simulink model "SystemComposer"  (R2023a)
settings: Solver=VariableStepAuto  StartTime=0.0  StopTime=10.0  RelTol=1e-3
settings Model: Creator=ycheb  LastModifiedBy=ycheb

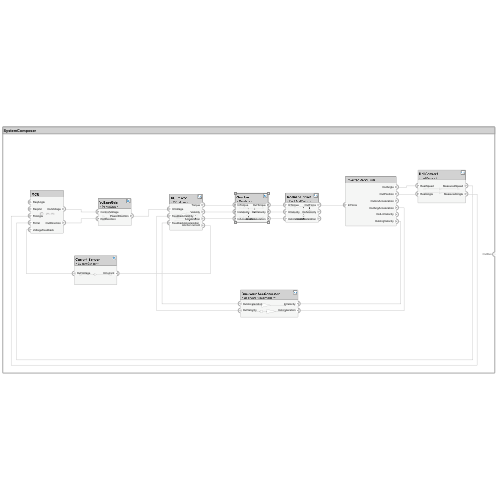
[thumbnail: Simulink's stored preview of the top-level diagram]
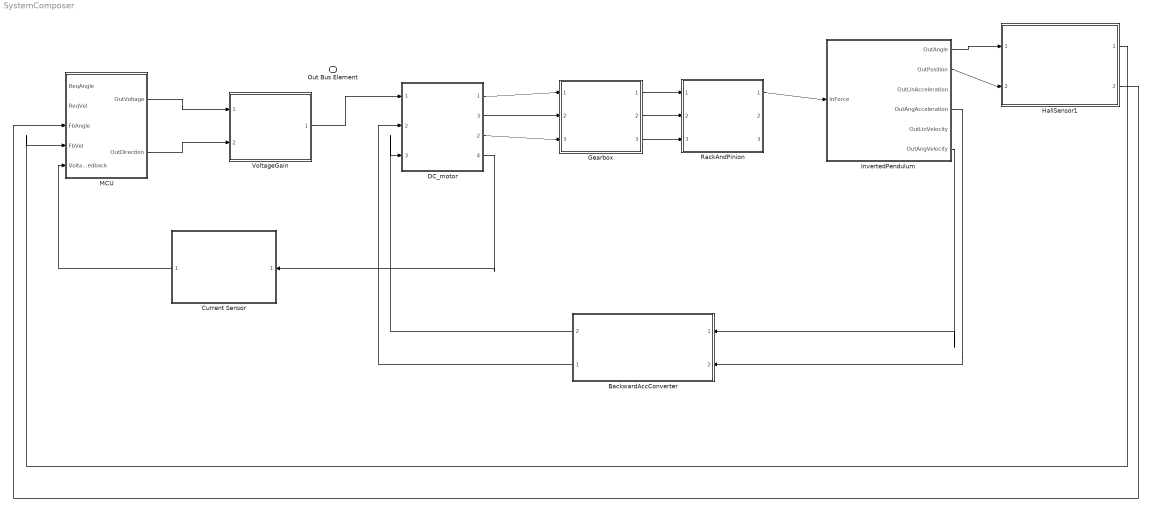
== system SystemComposer ==
  BackwardAccConverter : Subsystem  ReferencedSubsystem=BackwardAccConverter  i_gearbox=0  i_rail=0
      settings: PortSchema="{\"entries\":[{\"content\":{\"headerSize\":26,\"margin\":15,\"minimumSpacing\":25,\"sides\":[{\"content\":{\"connectorIds\":[\"Out2\",\"Out1\"]},\"type\":\"ConnectorPlacement.EquallySpacedRectSide\",\"uuid\":\"4580426d-ccc6-43cc-b0f4-903a280dd54a\"},{\"content\":{\"connectorIds\":[\"In1\",\"In2\"],\"side\":\"RIGHT\"},\"type\":\"ConnectorPlacement.EquallySpacedRectSide\",\"uuid\":\"b139a8af-3718-4301-b11f-f92378786662\"},{\"content\":{\"side\":\"TOP\"},\"type\":\"ConnectorPlacement.EquallySpacedRectSide\",\"uuid\":\"6cad6356-70f4-40af-85cc-1c4aec951e56\"}]},\"type\":\"ConnectorPlacement.EquallySpacedConnector\",\"uuid\":\"b6d7cb52-78ef-4ff8-a29a-dce0cd7ecabe\"}],\"packageUris\":[\"http://schema.mathworks.com/mf0/Connector/R2020b\"],\"version\":\"1.0\"}"
  Current Sensor : Subsystem  ReferencedSubsystem=CurrentSensor  R=0
      settings: PortSchema="{\"entries\":[{\"content\":{\"headerSize\":26,\"margin\":15,\"minimumSpacing\":25,\"sides\":[{\"content\":{\"connectorIds\":[\"Out1\"]},\"type\":\"ConnectorPlacement.EquallySpacedRectSide\",\"uuid\":\"1189f8f4-25dd-42ea-848e-97e302516e0e\"},{\"content\":{\"connectorIds\":[\"In1\"],\"side\":\"RIGHT\"},\"type\":\"ConnectorPlacement.EquallySpacedRectSide\",\"uuid\":\"7a8b9a95-7ade-4c5d-b769-aa776a1a8446\"},{\"content\":{\"side\":\"TOP\"},\"type\":\"ConnectorPlacement.EquallySpacedRectSide\",\"uuid\":\"ebb76304-2a77-452c-a318-4e5ff347d389\"}]},\"type\":\"ConnectorPlacement.EquallySpacedConnector\",\"uuid\":\"42e58dc7-ce24-4261-ad85-d72d6d49920a\"}],\"packageUris\":[\"http://schema.mathworks.com/mf0/Connector/R2020b\"],\"version\":\"1.0\"}"
  DC_motor : Subsystem  ReferencedSubsystem=DC_Motor  L=1  R=0  kw=0  km=0  J_motor=0  vis_friction_coef_motor=0
      settings: PortSchema="{\"entries\":[{\"content\":{\"headerSize\":26,\"margin\":15,\"minimumSpacing\":25,\"sides\":[{\"content\":{\"connectorIds\":[\"In1\",\"In2\",\"In3\"]},\"type\":\"ConnectorPlacement.EquallySpacedRectSide\",\"uuid\":\"195a28a2-a901-462e-beb9-5fc63a42afb4\"},{\"content\":{\"connectorIds\":[\"Out1\",\"Out3\",\"Out2\",\"Out4\"],\"side\":\"RIGHT\"},\"type\":\"ConnectorPlacement.EquallySpacedRectSide\",\"uuid\":\"0ccc545b-fa97-4bbe-bc7a-d14d9e9ad049\"},{\"content\":{\"side\":\"TOP\"},\"type\":\"ConnectorPlacement.EquallySpacedRectSide\",\"uuid\":\"58be0038-e581-4079-a9e4-051b8ced1df8\"}]},\"type\":\"ConnectorPlacement.EquallySpacedConnector\",\"uuid\":\"5194a1e3-6e8a-4730-ada4-e791e93f85f2\"}],\"packageUris\":[\"http://schema.mathworks.com/mf0/Connector/R2020b\"],\"version\":\"1.0\"}"
  Gearbox : Subsystem  ReferencedSubsystem=Gearbox  i=100  J_gear=2,4*10^-6  vis_friction_coef_gear=0.05
      settings: PortSchema="{\"entries\":[{\"content\":{\"headerSize\":26,\"margin\":15,\"minimumSpacing\":25,\"sides\":[{\"content\":{\"connectorIds\":[\"In1\",\"In2\",\"In3\"]},\"type\":\"ConnectorPlacement.EquallySpacedRectSide\",\"uuid\":\"4580426d-ccc6-43cc-b0f4-903a280dd54a\"},{\"content\":{\"connectorIds\":[\"Out1\",\"Out2\",\"Out3\"],\"side\":\"RIGHT\"},\"type\":\"ConnectorPlacement.EquallySpacedRectSide\",\"uuid\":\"b139a8af-3718-4301-b11f-f92378786662\"},{\"content\":{\"side\":\"TOP\"},\"type\":\"ConnectorPlacement.EquallySpacedRectSide\",\"uuid\":\"6cad6356-70f4-40af-85cc-1c4aec951e56\"}]},\"type\":\"ConnectorPlacement.EquallySpacedConnector\",\"uuid\":\"b6d7cb52-78ef-4ff8-a29a-dce0cd7ecabe\"}],\"packageUris\":[\"http://schema.mathworks.com/mf0/Connector/R2020b\"],\"version\":\"1.0\"}"
  HallSensor1 : Subsystem  ReferencedSubsystem=HallSensor
      settings: PortSchema="{\"entries\":[{\"content\":{\"headerSize\":26,\"margin\":15,\"minimumSpacing\":25,\"sides\":[{\"content\":{\"connectorIds\":[\"In1\",\"In2\"]},\"type\":\"ConnectorPlacement.EquallySpacedRectSide\",\"uuid\":\"d9e7e576-5a9b-43ea-8997-3be0b54a9a08\"},{\"content\":{\"connectorIds\":[\"Out1\",\"Out2\"],\"side\":\"RIGHT\"},\"type\":\"ConnectorPlacement.EquallySpacedRectSide\",\"uuid\":\"b8220865-259e-4734-b379-48897555c59f\"},{\"content\":{\"side\":\"TOP\"},\"type\":\"ConnectorPlacement.EquallySpacedRectSide\",\"uuid\":\"b1d688a9-3b35-4d53-b88e-55ef185f4acb\"}]},\"type\":\"ConnectorPlacement.EquallySpacedConnector\",\"uuid\":\"78f6d3ed-99d0-444d-b6d6-a0dd90eae3cb\"}],\"packageUris\":[\"http://schema.mathworks.com/mf0/Connector/R2020b\"],\"version\":\"1.0\"}"
  InvertedPendulum : Subsystem
      settings: PortSchema="{\"entries\":[{\"content\":{\"headerSize\":26,\"margin\":15,\"minimumSpacing\":25,\"sides\":[{\"content\":{\"connectorIds\":[\"In1\"]},\"type\":\"ConnectorPlacement.EquallySpacedRectSide\",\"uuid\":\"d9e7e576-5a9b-43ea-8997-3be0b54a9a08\"},{\"content\":{\"connectorIds\":[\"Out5\",\"Out6\",\"Out1\",\"Out2\",\"Out3\",\"Out4\"],\"side\":\"RIGHT\"},\"type\":\"ConnectorPlacement.EquallySpacedRectSide\",\"uuid\":\"b8220865-259e-4734-b379-48897555c59f\"},{\"content\":{\"side\":\"TOP\"},\"type\":\"ConnectorPlacement.EquallySpacedRectSide\",\"uuid\":\"b1d688a9-3b35-4d53-b88e-55ef185f4acb\"}]},\"type\":\"ConnectorPlacement.EquallySpacedConnector\",\"uuid\":\"78f6d3ed-99d0-444d-b6d6-a0dd90eae3cb\"}],\"packageUris\":[\"http://schema.mathworks.com/mf0/Connector/R2020b\"],\"version\":\"1.0\"}"
  MCU : Subsystem
      settings: PortSchema="{\"entries\":[{\"content\":{\"headerSize\":26,\"margin\":15,\"minimumSpacing\":25,\"sides\":[{\"content\":{\"connectorIds\":[\"In1\",\"In2\",\"In4\",\"In3\",\"In5\"]},\"type\":\"ConnectorPlacement.EquallySpacedRectSide\",\"uuid\":\"d9e7e576-5a9b-43ea-8997-3be0b54a9a08\"},{\"content\":{\"connectorIds\":[\"Out2\",\"Out1\"],\"side\":\"RIGHT\"},\"type\":\"ConnectorPlacement.EquallySpacedRectSide\",\"uuid\":\"b8220865-259e-4734-b379-48897555c59f\"},{\"content\":{\"side\":\"TOP\"},\"type\":\"ConnectorPlacement.EquallySpacedRectSide\",\"uuid\":\"b1d688a9-3b35-4d53-b88e-55ef185f4acb\"}]},\"type\":\"ConnectorPlacement.EquallySpacedConnector\",\"uuid\":\"78f6d3ed-99d0-444d-b6d6-a0dd90eae3cb\"}],\"packageUris\":[\"http://schema.mathworks.com/mf0/Connector/R2020b\"],\"version\":\"1.0\"}"
  RackAndPinion : Subsystem  ReferencedSubsystem=RackAndPinion  I_rail=0  m_rail=0  k_visco=0  i=0
      settings: PortSchema="{\"entries\":[{\"content\":{\"headerSize\":26,\"margin\":15,\"minimumSpacing\":25,\"sides\":[{\"content\":{\"connectorIds\":[\"In1\",\"In2\",\"In3\"]},\"type\":\"ConnectorPlacement.EquallySpacedRectSide\",\"uuid\":\"4580426d-ccc6-43cc-b0f4-903a280dd54a\"},{\"content\":{\"connectorIds\":[\"Out1\",\"Out2\",\"Out3\"],\"side\":\"RIGHT\"},\"type\":\"ConnectorPlacement.EquallySpacedRectSide\",\"uuid\":\"b139a8af-3718-4301-b11f-f92378786662\"},{\"content\":{\"side\":\"TOP\"},\"type\":\"ConnectorPlacement.EquallySpacedRectSide\",\"uuid\":\"6cad6356-70f4-40af-85cc-1c4aec951e56\"}]},\"type\":\"ConnectorPlacement.EquallySpacedConnector\",\"uuid\":\"b6d7cb52-78ef-4ff8-a29a-dce0cd7ecabe\"}],\"packageUris\":[\"http://schema.mathworks.com/mf0/Connector/R2020b\"],\"version\":\"1.0\"}"
  VoltageGain : Subsystem  ReferencedSubsystem=PowerGain  max_output_voltage=0  gain=0
      settings: PortSchema="{\"entries\":[{\"content\":{\"headerSize\":26,\"margin\":15,\"minimumSpacing\":25,\"sides\":[{\"content\":{\"connectorIds\":[\"In1\",\"In2\"]},\"type\":\"ConnectorPlacement.EquallySpacedRectSide\",\"uuid\":\"d9e7e576-5a9b-43ea-8997-3be0b54a9a08\"},{\"content\":{\"connectorIds\":[\"Out1\"],\"side\":\"RIGHT\"},\"type\":\"ConnectorPlacement.EquallySpacedRectSide\",\"uuid\":\"b8220865-259e-4734-b379-48897555c59f\"},{\"content\":{\"side\":\"TOP\"},\"type\":\"ConnectorPlacement.EquallySpacedRectSide\",\"uuid\":\"b1d688a9-3b35-4d53-b88e-55ef185f4acb\"}]},\"type\":\"ConnectorPlacement.EquallySpacedConnector\",\"uuid\":\"78f6d3ed-99d0-444d-b6d6-a0dd90eae3cb\"}],\"packageUris\":[\"http://schema.mathworks.com/mf0/Connector/R2020b\"],\"version\":\"1.0\"}"
  Out Bus Element : Outport  PortName=OutBus
  wires:
  InvertedPendulum/6(OutPosition) -> HallSensor1/2
  InvertedPendulum/5(OutAngle) -> HallSensor1/1
  HallSensor1/2 -> MCU/4(FbAngle)
  HallSensor1/1 -> MCU/3(FbVel)
  MCU/2(OutVoltage) -> VoltageGain/1
  MCU/1(OutDirection) -> VoltageGain/2
  Current Sensor/1 -> MCU/5(VoltageFeedback)
  DC_motor/1 -> Gearbox/1
  DC_motor/3 -> Gearbox/2
  DC_motor/2 -> Gearbox/3
  DC_motor/4 -> Current Sensor/1
  VoltageGain/1 -> DC_motor/1
  BackwardAccConverter/2 -> DC_motor/3
  BackwardAccConverter/1 -> DC_motor/2
  Gearbox/1 -> RackAndPinion/1
  Gearbox/2 -> RackAndPinion/2
  Gearbox/3 -> RackAndPinion/3
  RackAndPinion/1 -> InvertedPendulum/1(InForce)
  InvertedPendulum/2(OutAngAcceleration) -> BackwardAccConverter/2
  InvertedPendulum/4(OutAngVelocity) -> BackwardAccConverter/1

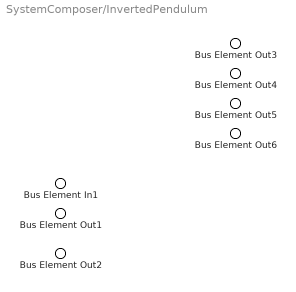
== system SystemComposer/InvertedPendulum ==
  Bus Element In1 : Inport  PortName=InForce
  Bus Element Out6 : Outport  PortName=OutLinAcceleration
  Bus Element Out5 : Outport  Port=2  PortName=OutAngAcceleration
  Bus Element Out4 : Outport  Port=3  PortName=OutLinVelocity
  Bus Element Out3 : Outport  Port=4  PortName=OutAngVelocity
  Bus Element Out1 : Outport  Port=5  PortName=OutAngle
  Bus Element Out2 : Outport  Port=6  PortName=OutPosition

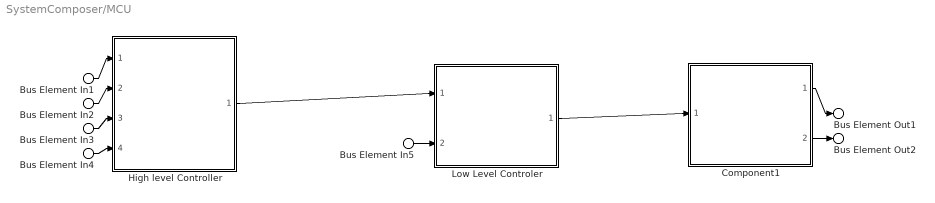
== system SystemComposer/MCU ==
  Bus Element In1 : Inport  PortName=ReqAngle
  Bus Element In2 : Inport  Port=2  PortName=ReqVel
  Bus Element In4 : Inport  Port=3  PortName=FbVel
  Bus Element In3 : Inport  Port=4  PortName=FbAngle
  Bus Element In5 : Inport  Port=5  PortName=VoltageFeedback
  Component1 : Subsystem  ReferencedSubsystem=ControlAdapter
      settings: PortSchema="{\"entries\":[{\"content\":{\"headerSize\":26,\"margin\":15,\"minimumSpacing\":25,\"sides\":[{\"content\":{\"connectorIds\":[\"In1\"]},\"type\":\"ConnectorPlacement.EquallySpacedRectSide\",\"uuid\":\"d9e7e576-5a9b-43ea-8997-3be0b54a9a08\"},{\"content\":{\"connectorIds\":[\"Out1\",\"Out2\"],\"side\":\"RIGHT\"},\"type\":\"ConnectorPlacement.EquallySpacedRectSide\",\"uuid\":\"b8220865-259e-4734-b379-48897555c59f\"},{\"content\":{\"side\":\"TOP\"},\"type\":\"ConnectorPlacement.EquallySpacedRectSide\",\"uuid\":\"b1d688a9-3b35-4d53-b88e-55ef185f4acb\"}]},\"type\":\"ConnectorPlacement.EquallySpacedConnector\",\"uuid\":\"78f6d3ed-99d0-444d-b6d6-a0dd90eae3cb\"}],\"packageUris\":[\"http://schema.mathworks.com/mf0/Connector/R2020b\"],\"version\":\"1.0\"}"
  High level Controller : Subsystem  ReferencedSubsystem=High_Level_Controller  k_i=0  k_p=0  k_d=0
      settings: PortSchema="{\"entries\":[{\"content\":{\"headerSize\":26,\"margin\":15,\"minimumSpacing\":25,\"sides\":[{\"content\":{\"connectorIds\":[\"In1\",\"In2\",\"In3\",\"In4\"]},\"type\":\"ConnectorPlacement.EquallySpacedRectSide\",\"uuid\":\"d9e7e576-5a9b-43ea-8997-3be0b54a9a08\"},{\"content\":{\"connectorIds\":[\"Out1\"],\"side\":\"RIGHT\"},\"type\":\"ConnectorPlacement.EquallySpacedRectSide\",\"uuid\":\"b8220865-259e-4734-b379-48897555c59f\"},{\"content\":{\"side\":\"TOP\"},\"type\":\"ConnectorPlacement.EquallySpacedRectSide\",\"uuid\":\"b1d688a9-3b35-4d53-b88e-55ef185f4acb\"}]},\"type\":\"ConnectorPlacement.EquallySpacedConnector\",\"uuid\":\"78f6d3ed-99d0-444d-b6d6-a0dd90eae3cb\"}],\"packageUris\":[\"http://schema.mathworks.com/mf0/Connector/R2020b\"],\"version\":\"1.0\"}"
  Low Level Controler : Subsystem  ReferencedSubsystem=LowLevelControler
      settings: PortSchema="{\"entries\":[{\"content\":{\"headerSize\":26,\"margin\":15,\"minimumSpacing\":25,\"sides\":[{\"content\":{\"connectorIds\":[\"In1\",\"In2\"]},\"type\":\"ConnectorPlacement.EquallySpacedRectSide\",\"uuid\":\"d9e7e576-5a9b-43ea-8997-3be0b54a9a08\"},{\"content\":{\"connectorIds\":[\"Out1\"],\"side\":\"RIGHT\"},\"type\":\"ConnectorPlacement.EquallySpacedRectSide\",\"uuid\":\"b8220865-259e-4734-b379-48897555c59f\"},{\"content\":{\"side\":\"TOP\"},\"type\":\"ConnectorPlacement.EquallySpacedRectSide\",\"uuid\":\"b1d688a9-3b35-4d53-b88e-55ef185f4acb\"}]},\"type\":\"ConnectorPlacement.EquallySpacedConnector\",\"uuid\":\"78f6d3ed-99d0-444d-b6d6-a0dd90eae3cb\"}],\"packageUris\":[\"http://schema.mathworks.com/mf0/Connector/R2020b\"],\"version\":\"1.0\"}"
  Bus Element Out2 : Outport  PortName=OutDirection
  Bus Element Out1 : Outport  Port=2  PortName=OutVoltage
  wires:
  Component1/1 -> Bus Element Out1/1
  Component1/2 -> Bus Element Out2/1
  Bus Element In5/1 -> Low Level Controler/2
  Low Level Controler/1 -> Component1/1
  High level Controller/1 -> Low Level Controler/1
  Bus Element In3/1 -> High level Controller/3
  Bus Element In4/1 -> High level Controller/4
  Bus Element In1/1 -> High level Controller/1
  Bus Element In2/1 -> High level Controller/2
